simulink model "crossroad_cs_old"  (R2021a)
settings: Solver=ode5  StartTime=0.0  StopTime=50  FixedStep=1/1000  RelTol=1e-3
PreLoadFcn:
  | mbxruntime.callbacks.PreLoadFcn(bdroot);
PostLoadFcn:
  | mbxruntime.callbacks.PostLoadFcn(bdroot);
InitFcn:
  | mbxruntime.callbacks.InitFcn(bdroot);
StartFcn:
  | mbxruntime.callbacks.StartFcn(bdroot);
StopFcn:
  | mbxruntime.callbacks.StopFcn(bdroot);
model workspace: external: MAT-File .\crossroad_cs_hws.mat (data not in the file)
values from neighbouring files (symbols this model uses):
  c_factor = 43.75    [emplanner_init.m]
  cf = -175016    [emplanner_init.m]
  cr = -130634    [emplanner_init.m]
  KD_PID_distance = 0.0    (= 0)    [emplanner_init.m]
  KD_PID_speed = 0    [emplanner_init.m]
  KI_PID_distance = 0.0    (= 0)    [emplanner_init.m]
  KI_PID_speed = 0    [emplanner_init.m]
  KP_PID_distance = 0.5    [emplanner_init.m]
  KP_PID_speed = 1.8    [emplanner_init.m]
  la = 1.265    [emplanner_init.m]
  lb = 2.947-1.265    (= 1.682)    [emplanner_init.m]
  LQR_K1 = k(:,1)'    [emplanner_init.m]
  LQR_K2 = k(:,2)'    [emplanner_init.m]
  LQR_K3 = k(:,3)'    [emplanner_init.m]
  LQR_K4 = k(:,4)'    [emplanner_init.m]
  m = 2020    [emplanner_init.m]
  my_global_path_x = [0.4409 0.940746626271 1.44028225507 1.93950267328 2.43840536558 2.93698884522 3.43525224935 3.93319509352 4.43081712279 4.92811822143 5.42509835808 5.92175755256 ... (6001 elements, 6001x1)]    [my_global_path.mat]    (also in my_global_path_200.mat = [0.4409 0.940746626271 1.44028225507 1.93950267328 2.4384053)
  my_global_path_y = [58.2244 58.2243999975 58.2243999675 58.2243998683 58.224399668 58.2243993499 58.2243989099 58.2243983526 58.2243976886 58.2243969324 58.2243961011 58.2243952132 ... (6001 elements, 6001x1)]    [my_global_path.mat]    (also in my_global_path_200.mat = [58.2244 58.2243999975 58.2243999675 58.2243998683 58.224399)
  rack_displacement = [-39.14 , -37.2 , -35.29 , -33.43 , -31.6 , -29.81 , -28.06 , -26.34 , -24.66 ,      -23.01 , -21.38 , -19.79 , -18.23 , -16.69 , -15.18 , -13.7 , -12.23 , -10.8 , -9.38 , -7.98 ,     -6.61 , -5.25 , -3.91 , -2.59 , -1.29 , 0 , 1.27 , 2.54 , 3.78 , 5.02 , 6.24 , 7.46 , 8.66 ,      9.86 , 11.05 , 12.24 , 13.41 , 14.59 , 15.76 , 16.92 , 18.09 , 19.25 , 20.42 , 21.59 , 22.76 ,      23.93 , 25.11 , 26 ...(+26 chars)    [emplanner_init.m]
  right_wheel_ground = [-70 ,-67.2 , -64.4 , -61.6 , -58.8 , -56 , -53.2 , -50.4 , -47.6 , -44.8 , -42 ,      -39.2 , -36.4 , -33.6 , -30.8 , -28 , -25.2 , -22.4 , -19.6 , -16.8 , -14 , -11.2 , -8.4 , -5.6 ,      -2.8 , 0 , 2.8 , 5.6 , 8.4 , 11.2 , 14 , 16.8 , 19.6 , 22.4 , 25.2 , 28 , 30.8 , 33.6 , 36.4 ,      39.2 , 42 , 44.8 , 47.6 , 50.4 , 53.2 , 56 , 58.8 , 61.6 , 64.4 , 67.2 , 70 ]    [emplanner_init.m]
  vx_break_point = zeros(1,5000)    [emplanner_init.m]
undefined symbols (not defined in the file or in its folder): aubr, DiscIntNeverNeededParam, tablebr, vubr
libraries: PreScanSimulinkLibrary x11, Solver_SF x1
(part 2 of 8)

== system crossroad_cs_old/STATE_Box_4_bus ==
  STATE_Box_4_bus : Inport  Tag=inport/StatePort  OutDataTypeStr=Bus: PRESCAN_STATEACTUATORDATA  PortDimensions=1  SampleTime=50/1000  BusOutputAsStruct=on
  Actuator : S-Function  FunctionName=sfun_StateActuator  Parameters=UniqueID, TimeStep  SFunctionDeploymentMode=off  EnableBusSupport=off  mask(PreScan Sink Block: State){UniqueID=745, TimeStep=50/1000}
      mask prompts: UniqueID "Auto-Assigned: Unique ID"; TimeStep "Auto-Assigned: Upload Period [s]"
      mask help:
      | The Actor State contains a vector signal of size (9x1), containing the following signals:
      |
      | -  Position    	(x,y,z)             	[m]
      | -  Velocity    	(vx,vy,vz)         	[m/s]
      | -  Angles       	(Roll, Pitch, Yaw)	[rad]
      |
      | The Actor state is defined in the global axis system.
      | The state is superponed on the Initial position defined in the GUI.
      |
      | For more information, please click Help.
      mask Help: eval('openHelp(222)')
      mask Display: image(imread('State.png'))
  wires:
  STATE_Box_4_bus/1 -> Actuator/1

== system crossroad_cs_old/Synchronizer ==
  Bus Selector1 : BusSelector  OutputSignals=FederateStopped
  Stop Simulation : Stop
  sfun_Synchronizer : S-Function  FunctionName=sfun_Synchronizer  Parameters=SampleTime  SFunctionDeploymentMode=off  EnableBusSupport=off  mask(Legacy Function){SFunctionSpec=void prescan_synchronizer_outputFcn(void ** work1, PRESCAN_SYNCHRONIZEDATA y1[1]), SampleTime=TimeStep, ShowSpec=on}
      mask prompts: SampleTime "Sample time (-1 for inherited):"; ShowSpec "Display function specification"
      mask help:
      | This block allows you to call the legacy functions specified by the following Legacy Code Tool definition:
      | def.SFunctionName = 'sfun_Synchronizer';
      | def.OutputFcnSpec = 'void prescan_synchronizer_outputFcn(void ** work1, PRESCAN_SYNCHRONIZEDATA y1[1])';
      | def.StartFcnSpec = 'void prescan_synchronizer_startFcn(void ** work1)';
      | def.TerminateFcnSpec = 'void prescan_synchronizer_terminateFcn(void ** work1)';
      | def.HeaderFiles = {'prescan_synchronizer_data.h'};
      | def.HostLibFiles = {'sensorinterfaced.lib'};
      | def.IncPaths = {'src', 'C:\prescandev\vislibrary\vis\..\pimp\include\sensors\InterfaceRTW'};
      | def.SrcPaths = {'src'};
      | def.LibPaths = {'C:\\prescandev\\vislibrary_build\lib'};
      | def.SampleTime = 'parameterized';
      | def.Options.language = 'C';
      mask Help: <p>This block was generated automatically by the Legacy Code Tool. For detailed help on this tool, call<a href="matlab:legacy_code('help')"> legacy_code('help')</a>.</p>
      mask Callback ShowSpec:
      | if strcmp(get_param(gcbh, 'ShowSpec'), 'on')
      |   set_param(gcbh, 'MaskDisplay', sprintf('fprintf(''%s'');', get_param(gcbh, 'SFunctionSpec')));
      | else
      |   set_param(gcbh, 'MaskDisplay', sprintf('fprintf(''%s'');', get_param(gcbh, 'FunctionName')));
      | end
      mask Display: fprintf('void prescan_synchronizer_outputFcn(void ** work1, PRESCAN_SYNCHRONIZEDATA y1[1])');
  wires:
  Bus Selector1/1 -> Stop Simulation/1  "<FederateStopped>"
  sfun_Synchronizer/1 -> Bus Selector1/1

== system crossroad_cs_old/Audi_A8_Sedan_1/AIR_1_Demux ==
  AIR : Inport
  Activate_Switch : Subsystem
      mask Display: text(5,10,'')
  Bus Selector : BusSelector  OutputSignals=DATA.Range,DATA.Azimuth,DATA.Elevation,DATA.ID,DATA.Velocity,DATA.Heading
  Data Type Conversion : DataTypeConversion  OutDataTypeStr=double
  For Iterator : ForIterator  ResetStates=reset  IterationLimit=detectableObjects
  Selector : Selector  InputPortWidth=detectableObjects  IndexOptions=Index vector (port)  Indices=[1 3]  OutputSizes=1
  Signal2ArrayOfSignals1 : Subsystem  mask{VECTORLENGTH=detectableObjects}
      mask prompts: VECTORLENGTH "Length of vector"
  Signal2ArrayOfSignals2 : Subsystem  mask{VECTORLENGTH=detectableObjects}
      mask prompts: VECTORLENGTH "Length of vector"
  Signal2ArrayOfSignals3 : Subsystem  mask{VECTORLENGTH=detectableObjects}
      mask prompts: VECTORLENGTH "Length of vector"
  Signal2ArrayOfSignals4 : Subsystem  mask{VECTORLENGTH=detectableObjects}
      mask prompts: VECTORLENGTH "Length of vector"
  Signal2ArrayOfSignals5 : Subsystem  mask{VECTORLENGTH=detectableObjects}
      mask prompts: VECTORLENGTH "Length of vector"
  Signal2ArrayOfSignals6 : Subsystem  mask{VECTORLENGTH=detectableObjects}
      mask prompts: VECTORLENGTH "Length of vector"
  Range [m] : Outport
  Azimuth [deg] : Outport  Port=2
  Elevation [deg] : Outport  Port=3
  ID [-] : Outport  Port=4
  Velocity [m/s] : Outport  Port=5
  Heading [deg] : Outport  Port=6
  wires:
  Data Type Conversion/1 -> ID [-]/1
  Bus Selector/6 -> Signal2ArrayOfSignals6/2(Element)  "<Heading>"
  Signal2ArrayOfSignals6/1(ArrayofElements) -> Activate_Switch/2(Heading)
  Bus Selector/5 -> Signal2ArrayOfSignals5/2(Element)  "<Velocity>"
  Signal2ArrayOfSignals5/1(ArrayofElements) -> Velocity [m/s]/1
  Bus Selector/4 -> Signal2ArrayOfSignals4/2(Element)  "<ID>"
  Signal2ArrayOfSignals4/1(ArrayofElements) -> Data Type Conversion/1, Activate_Switch/1(BeamID)
  Bus Selector/3 -> Signal2ArrayOfSignals3/2(Element)  "<Elevation>"
  Signal2ArrayOfSignals3/1(ArrayofElements) -> Elevation [deg]/1
  Bus Selector/2 -> Signal2ArrayOfSignals1/2(Element)  "<Azimuth>"
  Signal2ArrayOfSignals1/1(ArrayofElements) -> Azimuth [deg]/1
  Signal2ArrayOfSignals2/1(ArrayofElements) -> Range [m]/1
  Bus Selector/1 -> Signal2ArrayOfSignals2/2(Element)  "<Range>"
  Selector/1 -> Bus Selector/1
  For Iterator/1 -> Signal2ArrayOfSignals6/1(LoopIndex), Signal2ArrayOfSignals5/1(LoopIndex), Signal2ArrayOfSignals4/1(LoopIndex), Signal2ArrayOfSignals3/1(LoopIndex), Signal2ArrayOfSignals1/1(LoopIndex), Signal2ArrayOfSignals2/1(LoopIndex), Selector/2
  AIR/1 -> Selector/1
  Activate_Switch/1(On/Off) -> Heading [deg]/1

== system crossroad_cs_old/Audi_A8_Sedan_1/Dynamics_UserSpecified ==
  note: For state mode 'Dynamic' positions
      | are not taken into account, as they
      | are computed by integrating velocity.
      | Click annotation for Help.
  steer_sw : Inport
  throttle : Inport  Port=2
  brake : Inport  Port=3
  CarSim S-Function2 : Solver_SF/CarSim S-Function  Priority=1  SIMFILE=D:\CARSIM2019.1\DynamicModel\simfile.sim
  CarSim2PreScanSTATE : Subsystem  Tag=CarSim2PreScanSTATE  mask(CarSim2PreScan:){z0=0}
      mask prompts: z0 "PreScan Actor initial COG z-position wrt GLOBAL axis system [m]"
      mask help: This block converts the outputs coming from the CarSim block into consistent PreScan signals.
  Constant : Constant  Value=ones(1,8)*1
  Ground : Ground
  Ground1 : Ground
  Mux : Mux  Inputs=[1 1 1 12 8]
  MuxState : Subsystem  Tag=mux/State  mask(Empty Dynamics State Block){positioningmode=on, TimeStep=1/1000}
      mask prompts: positioningmode "Positioning Mode"; TimeStep "Auto Assigned: Time Step [s]"
      mask help:
      | Build the state of an actor based on user input.
      | The user can either use positioning mode or dynamics mode.
      | - When using positioning mode the position and orientation of the actor are set directly based on the input. Expected input is relative to the initial position and orientation of the actor. It's also possible to specify the velocity of the actor, though this input isn't used, only passed on.
      | - When using dynamics mode the position input is ignored. Expected input is velocity and orientation. The velocity is relative the current orientation of the actor, while orientation is relative to its initial orientation. The position of the actor is calculated based on the velocity and orientation given.
      settings: DeleteFcn=PreScanBlockDeleteFcn;
  STATE_Audi_A8_Sedan_1 : Subsystem  Tag=mux/StatePort  Priority=0  LoadFcn=load PrescanStateActuatorData  mask(PreScan Sink Block: State){x0=3.6384, y0=57.8912, z0=0.55, Roll0=0, Pitch0=0, Yaw0=0, TimeStep=1/1000}
      mask prompts: x0 "Ini x-position VEHICLE wrt GLOBAL axis system [m]"; y0 "Ini y-position VEHICLE wrt GLOBAL axis system [m]"; z0 "Ini z-position VEHICLE wrt GLOBAL axis system [m]"; Roll0 "Ini roll-angle BODY wrt VEHICLE axis system [deg]"; Pitch0 "Ini pitch-angle BODY wrt VEHICLE axis system [deg]"; Yaw0 "Ini yaw-angle VEHICLE wrt GLOBAL axis system [deg]"; TimeStep "Auto-Assigned: Upload Period [s]"
      mask help:
      | The Actor State contains a vector signal of size (9x1), containing the following signals:
      |
      | -  Position                  (x,y,z)                                     [m]
      | -  Velocity                  (vx,vy,vz)                               [m/s]
      | -  Angles                    (Roll, Pitch, Yaw)                   [rad]
      |
      | The Actor state is defined in the global axis system.
      | The state is superponed on the Initial position defined in the GUI.
      |
      | For more information, please click Help.
      settings: DeleteFcn=PreScanBlockDeleteFcn;
      mask Help: eval('openHelp(222)')
      mask Display: image(imread('State.png'))
  Scope : Scope
  State : Outport
  vx : Outport  Port=2
  vy : Outport  Port=3
  ax : Outport  Port=4
  ay : Outport  Port=5
  wires:
  Ground/1 -> Mux/4
  brake/1 -> Mux/3
  steer_sw/1 -> Mux/1
  Constant/1 -> Mux/5
  throttle/1 -> Mux/2
  CarSim S-Function2/1 -> CarSim2PreScanSTATE/1(CarSim_In)
  CarSim2PreScanSTATE/7(R [rad]) -> MuxState/7(R [rad])
  CarSim2PreScanSTATE/9(Y [rad]) -> MuxState/9(Y [rad])
  CarSim2PreScanSTATE/11(ay[m/s^2]) -> ay/1
  CarSim2PreScanSTATE/2(y [m]) -> MuxState/2(y [m])
  CarSim2PreScanSTATE/6(dz [m/s]) -> MuxState/6(dz [m/s])
  CarSim2PreScanSTATE/10(ax[m/s^2]) -> ax/1
  CarSim2PreScanSTATE/1(x [m]) -> Scope/1, MuxState/1(x [m])
  CarSim2PreScanSTATE/4(dx [m/s]) -> vx/1, MuxState/4(dx [m/s])
  CarSim2PreScanSTATE/8(P [rad]) -> MuxState/8(P [rad])
  CarSim2PreScanSTATE/3(z [m]) -> MuxState/3(z [m])
  CarSim2PreScanSTATE/5(dy [m/s]) -> vy/1, MuxState/5(dy [m/s])
  MuxState/1(state) -> State/1, STATE_Audi_A8_Sedan_1/1(State)
  Mux/1 -> CarSim S-Function2/1
  Ground1/1 -> ?
  STATE_Audi_A8_Sedan_1/1(StateBus) -> ?

== system crossroad_cs_old/Audi_A8_Sedan_1/SELF_Demux ==
  SELF : Inport  OutDataTypeStr=Bus: PRESCAN_SELFSENSORDATA
  Bus Selector : BusSelector  OutputSignals=PositionX,PositionY,PositionZ,OrientationRoll,OrientationPitch,OrientationYaw,Velocity,Yaw_rate,Lat,Long,Alt
  Demux2 : Demux  Outputs=3
  Gain : Gain  Gain=180/pi
  Gain1 : Gain  Gain=180/pi
  Vector Concatenate1 : Concatenate  NumInputs=3
  compas converter : Subsystem
  x [m] : Outport
  y [m] : Outport  Port=2
  z [m] : Outport  Port=3
  rotx [deg] : Outport  Port=4
  roty [deg] : Outport  Port=5
  rotz [deg] : Outport  Port=6
  GPS lat [deg] : Outport  Port=7
  GPS long [deg] : Outport  Port=8
  GPS alt [m] : Outport  Port=9
  velocity [m/s] : Outport  Port=10
  heading [deg] : Outport  Port=11
  yaw rate [deg/s] : Outport  Port=12
  wires:
  Bus Selector/11 -> GPS alt [m]/1  "<Alt>"
  Bus Selector/10 -> GPS long [deg]/1  "<Long>"
  Bus Selector/9 -> GPS lat [deg]/1  "<Lat>"
  Bus Selector/8 -> Gain1/1  "<Yaw_rate>"
  Bus Selector/6 -> compas converter/1(rotz [rad]), Vector Concatenate1/3  "<OrientationYaw>"
  Bus Selector/5 -> Vector Concatenate1/2  "<OrientationPitch>"
  Bus Selector/4 -> Vector Concatenate1/1  "<OrientationRoll>"
  Vector Concatenate1/1 -> Gain/1
  Bus Selector/3 -> z [m]/1  "<PositionZ>"
  SELF/1 -> Bus Selector/1
  Gain/1 -> Demux2/1
  Demux2/1 -> rotx [deg]/1
  Demux2/2 -> roty [deg]/1
  Demux2/3 -> rotz [deg]/1
  compas converter/1(heading [deg]) -> heading [deg]/1
  Gain1/1 -> yaw rate [deg/s]/1
  Bus Selector/1 -> x [m]/1  "<PositionX>"
  Bus Selector/2 -> y [m]/1  "<PositionY>"
  Bus Selector/7 -> velocity [m/s]/1  "<Velocity>"

== system crossroad_cs_old/Audi_A8_Sedan_1/STATE_Audi_A8_Sedan_1 ==
  State : Inport  SampleTime=TimeStep
  Bus Creator : BusCreator  Inputs=15  OutDataTypeStr=Bus: PRESCAN_STATEACTUATORDATA  NonVirtualBus=on
  Constant : Constant  Value=0
  Demux : Demux  Outputs=15
  Mux : Mux  Inputs=3
  Mux1 : Mux  Inputs=3
  Mux2 : Mux  Inputs=3
  iniBODYAngles wrtVEH [rad] : Constant  Value=Roll0  SampleTime=TimeStep
  iniBODYAngles wrtVEH [rad]1 : Constant  Value=Pitch0  SampleTime=TimeStep
  iniVEHAngles wrtGLOB [rad] : Constant  Value=Yaw0  SampleTime=TimeStep
  iniVEHposition wrtGLOB [m] : Constant  Value=x0  SampleTime=TimeStep
  iniVEHposition wrtGLOB [m]1 : Constant  Value=y0  SampleTime=TimeStep
  iniVEHposition wrtGLOB [m]2 : Constant  Value=z0  SampleTime=TimeStep
  state2FullState : PreScanSimulinkLibrary/state2FullState  SystemSampleTime=-1  VariantActivationTime=update diagram  Latency=0  AutoFrameSizeCalculation=off
  StateBus : Outport  OutDataTypeStr=Bus: PRESCAN_STATEACTUATORDATA
  wires:
  Mux2/1 -> state2FullState/4
  iniVEHAngles wrtGLOB [rad]/1 -> Mux2/3
  Mux1/1 -> state2FullState/3
  Constant/1 -> Mux2/1, Mux2/2, Mux1/3
  iniBODYAngles wrtVEH [rad]1/1 -> Mux1/2
  iniBODYAngles wrtVEH [rad]/1 -> Mux1/1
  Mux/1 -> state2FullState/2
  iniVEHposition wrtGLOB [m]2/1 -> Mux/3
  iniVEHposition wrtGLOB [m]/1 -> Mux/1
  iniVEHposition wrtGLOB [m]1/1 -> Mux/2
  Demux/15 -> Bus Creator/15  "AngularVelocityYaw"
  Demux/14 -> Bus Creator/14  "AngularVelocityPitch"
  Demux/13 -> Bus Creator/13  "AngularVelocityRoll"
  Demux/12 -> Bus Creator/12  "OrientationYaw"
  Demux/11 -> Bus Creator/11  "OrientationPitch"
  Demux/10 -> Bus Creator/10  "OrientationRoll"
  Demux/9 -> Bus Creator/9  "AccelerationZ"
  Demux/8 -> Bus Creator/8  "AccelerationY"
  Demux/7 -> Bus Creator/7  "AccelerationX"
  Demux/6 -> Bus Creator/6  "VelocityZ"
  Demux/5 -> Bus Creator/5  "VelocityY"
  Demux/4 -> Bus Creator/4  "VelocityX"
  Demux/3 -> Bus Creator/3  "PositionZ"
  Demux/2 -> Bus Creator/2  "PositionY"
  Demux/1 -> Bus Creator/1  "PositionX"
  state2FullState/1 -> Demux/1
  State/1 -> state2FullState/1
  Bus Creator/1 -> StateBus/1

== system crossroad_cs_old/Audi_A8_Sedan_1/control module1 ==
  location_info : Inport
  planning_result : Inport  Port=2
  control_predict_time[s] : Inport  Port=3
  current_time : Inport  Port=4
  Trigger : TriggerPort  TriggerType=function-call  VariantControl=Variant  PortDimensions=1
  Bus Selector : BusSelector  OutputSignals=trajectory_x_gcs,trajectory_y_gcs,trajectory_heading_gcs,trajectory_kappa_gcs,trajectory_speed_gcs,trajectory_accel_gcs,trajectory_time_gcs
  Bus Selector1 : BusSelector  OutputSignals=host_x,host_y,host_heading_xy,host_vx,host_vy,host_yawrate,host_speed
  MATLAB Function : MATLAB Function  TreatAsAtomicUnit=on
  control main : Subsystem
  lateral_steer_sw : Outport
  throttle : Outport  Port=2
  brake : Outport  Port=3
  debug_control : Outport  Port=4
  wires:
  Bus Selector1/5 -> control main/5(host_vy[m/s])  "<host_vy>"
  Bus Selector1/4 -> control main/4(host_vx[m/s])  "<host_vx>"
  Bus Selector1/2 -> control main/2(host_y[m])  "<host_y>"
  Bus Selector1/7 -> control main/7(host_speed[m/s])  "<host_speed>"
  control main/2(throttle) -> throttle/1
  Bus Selector1/1 -> control main/1(host_x[m])  "<host_x>"
  Bus Selector1/6 -> control main/6(host_yawrate[rad/s])  "<host_yawrate>"
  Bus Selector1/3 -> control main/3(host_heading_xy[rad])  "<host_heading_xy>"
  location_info/1 -> Bus Selector1/1
  control_predict_time[s]/1 -> control main/14(control_predict_time[s])
  control main/4(debug_control) -> debug_control/1
  control main/1(lateral_steer_sw) -> lateral_steer_sw/1
  control main/3(brake) -> brake/1
  MATLAB Function/6(ar) -> control main/13(accelerate_desire[m/s^2])
  MATLAB Function/5(vr) -> control main/12(speed_desire[m/s])
  MATLAB Function/4(kappar) -> control main/11(kappar_desire[m^-1])
  MATLAB Function/3(thetar) -> control main/10(thetar_desire[rad])
  MATLAB Function/2(yr) -> control main/9(yr_desire[m])
  MATLAB Function/1(xr) -> control main/8(xr_desire[m])
  current_time/1 -> MATLAB Function/8(current_time)
  planning_result/1 -> Bus Selector/1
  Bus Selector/1 -> [trajecotory_x]  "<trajectory_x_gcs>"
  Bus Selector/2 -> [trajecotory_y]  "<trajectory_y_gcs>"
  Bus Selector/3 -> [trajecotory_heading]  "<trajectory_heading_gcs>"
  Bus Selector/4 -> [trajecotory_kappa]  "<trajectory_kappa_gcs>"
  Bus Selector/5 -> [trajecotory_speed]  "<trajectory_speed_gcs>"
  Bus Selector/6 -> [trajecotory_accel]  "<trajectory_accel_gcs>"
  Bus Selector/7 -> [trajecotory_time]  "<trajectory_time_gcs>"
  [trajecotory_time] -> MATLAB Function/7(trajectory_time)
  [trajecotory_accel] -> MATLAB Function/6(trajectory_accel)
  [trajecotory_speed] -> MATLAB Function/5(trajectory_speed)
  [trajecotory_kappa] -> MATLAB Function/4(trajectory_kappa)
  [trajecotory_heading] -> MATLAB Function/3(trajectory_heading)
  [trajecotory_y] -> MATLAB Function/2(trajectory_y)
  [trajecotory_x] -> MATLAB Function/1(trajectory_x)

== system crossroad_cs_old/Audi_A8_Sedan_1/decision&planning module ==
  location info : Inport
  routine info : Inport  Port=2
  perception info : Inport  Port=3
  pre planning info : Inport  Port=4
  current time : Inport  Port=5
  Trigger : TriggerPort  TriggerType=function-call  VariantControl=Variant  PortDimensions=1
  Bus Selector : BusSelector  OutputSignals=host_x,host_y,host_heading_xy,host_vx,host_vy,host_yawrate,host_speed
  Bus Selector1 : BusSelector  OutputSignals=referenceline_x,referenceline_y,referenceline_heading,referenceline_kappa
  EM Planner : Subsystem
  referenceline provider : Subsystem
  planning_result : Outport
  wires:
  [planning_result] -> planning_result/1
  routine info/1 -> referenceline provider/2(routine info)
  location info/1 -> EM Planner/2(location info), Bus Selector/1, referenceline provider/1(location info)
  Bus Selector/7 -> [host_speed]  "<host_speed>"
  Bus Selector/1 -> [host_x]  "<host_x>"
  Bus Selector/3 -> [host_heading_xy]  "<host_heading_xy>"
  Bus Selector/4 -> [host_vx]  "<host_vx>"
  Bus Selector/5 -> [host_vy]  "<host_vy>"
  Bus Selector/2 -> [host_y]  "<host_y>"
  Bus Selector/6 -> [host_yawrate]  "<host_yawrate>"
  referenceline provider/1(referenceline info) -> EM Planner/1(referenceline info), [referenceline_info]
  referenceline provider/2(debug referenceline) -> [debug_referenceline]
  [referenceline_info] -> Bus Selector1/1
  Bus Selector1/1 -> [referenceline_x]  "<referenceline_x>"
  Bus Selector1/2 -> [referenceline_y]  "<referenceline_y>"
  Bus Selector1/3 -> [referenceline_heading]  "<referenceline_heading>"
  Bus Selector1/4 -> [referenceline_kappa]  "<referenceline_kappa>"
  perception info/1 -> EM Planner/3(perception info)
  pre planning info/1 -> EM Planner/4(pre_planning info)
  current time/1 -> EM Planner/5(current time)
  EM Planner/1(EM Planner result) -> [planning_result]

== system crossroad_cs_old/Audi_A8_Sedan_1/location module ==
  host_x[m] : Inport
  host_y[m] : Inport  Port=2
  host_heading_xy[rad] : Inport  Port=3
  host_vx[m/s] : Inport  Port=4
  host_vy[m/s] : Inport  Port=5
  host_yawrate[rad/s] : Inport  Port=6
  host_speed[m/s] : Inport  Port=7
  host_ax[m/s2] : Inport  Port=8
  host_ay[m/s2] : Inport  Port=9
  Bus Creator : BusCreator  Inputs=9
  location info : Outport
  wires:
  host_yawrate[rad/s]/1 -> Bus Creator/6
  host_vy[m/s]/1 -> Bus Creator/5
  host_heading_xy[rad]/1 -> Bus Creator/3
  host_speed[m/s]/1 -> Bus Creator/7
  Bus Creator/1 -> location info/1
  host_y[m]/1 -> Bus Creator/2
  host_x[m]/1 -> Bus Creator/1
  host_vx[m/s]/1 -> Bus Creator/4
  host_ax[m/s2]/1 -> Bus Creator/8
  host_ay[m/s2]/1 -> Bus Creator/9

== system crossroad_cs_old/Audi_A8_Sedan_1/perception module ==
  location info : Inport
  obs range : Inport  Port=2
  obs theta : Inport  Port=3
  obs velocity : Inport  Port=4
  obs heading : Inport  Port=5
  Bus Creator : BusCreator  Inputs=4
  Bus Selector : BusSelector  OutputSignals=host_x,host_y,host_heading_xy
  MATLAB Function : MATLAB Function  TreatAsAtomicUnit=on
  perception info : Outport
  wires:
  location info/1 -> Bus Selector/1
  Bus Selector/1 -> [host_x]  "<host_x>"
  Bus Selector/2 -> [host_y]  "<host_y>"
  Bus Selector/3 -> [host_heading_xy]  "<host_heading_xy>"
  obs range/1 -> [obs_range]
  obs theta/1 -> [obs_theta]
  obs velocity/1 -> [obs_velocity]
  obs heading/1 -> [obs_heading]
  [host_x] -> MATLAB Function/1(host_x)
  [host_y] -> MATLAB Function/2(host_y)
  [host_heading_xy] -> MATLAB Function/3(host_heading_xy)
  [obs_range] -> MATLAB Function/4(obs_range)
  [obs_theta] -> MATLAB Function/5(obs_theta)
  [obs_velocity] -> MATLAB Function/6(obs_velocity)
  [obs_heading] -> MATLAB Function/7(obs_velocity_heading)
  MATLAB Function/1(obs_x_set_gcs) -> [obs_x_set_gcs]
  MATLAB Function/2(obs_y_set_gcs) -> [obs_y_set_gcs]
  MATLAB Function/3(obs_velocity_set_gcs) -> [obs_velocity_set_gcs]
  MATLAB Function/4(obs_heading_set_gcs) -> [obs_heading_set_gcs]
  Bus Creator/1 -> perception info/1
  [obs_x_set_gcs] -> Bus Creator/1  "obs_x_set_gcs"
  [obs_y_set_gcs] -> Bus Creator/2  "obs_y_set_gcs"
  [obs_velocity_set_gcs] -> Bus Creator/3  "obs_velocity_set_gcs"
  [obs_heading_set_gcs] -> Bus Creator/4  "obs_heading_set_gcs"

== system crossroad_cs_old/Audi_A8_Sedan_1/routine module ==
  Bus Creator : BusCreator  Inputs=2
  Constant : Constant  Value=my_global_path_x
  Constant1 : Constant  Value=my_global_path_y
  global_path_info : Outport
  wires:
  Constant1/1 -> [global_path_y]
  Constant/1 -> [global_path_x]
  [global_path_x] -> Bus Creator/1  "global_path_x"
  [global_path_y] -> Bus Creator/2  "global_path_y"
  Bus Creator/1 -> global_path_info/1

== system crossroad_cs_old/Box_1/Dynamics_Empty ==
  note: For state mode 'Dynamic' positions
      | are not taken into account, as they
      | are computed by integrating velocity.
      | Click annotation for Help.
  Ground_{1..9} (9 alike) : Ground
  MuxState : Subsystem  Tag=mux/State  mask(Empty Dynamics State Block){positioningmode=on, TimeStep=1/1000}
      mask prompts: positioningmode "Positioning Mode"; TimeStep "Auto Assigned: Time Step [s]"
      mask help:
      | Build the state of an actor based on user input.
      | The user can either use positioning mode or dynamics mode.
      | - When using positioning mode the position and orientation of the actor are set directly based on the input. Expected input is relative to the initial position and orientation of the actor. It's also possible to specify the velocity of the actor, though this input isn't used, only passed on.
      | - When using dynamics mode the position input is ignored. Expected input is velocity and orientation. The velocity is relative the current orientation of the actor, while orientation is relative to its initial orientation. The position of the actor is calculated based on the velocity and orientation given.
      settings: DeleteFcn=PreScanBlockDeleteFcn;
  STATE_Box_1 : Subsystem  Tag=mux/StatePort  Priority=0  LoadFcn=load PrescanStateActuatorData  mask(PreScan Sink Block: State){x0=97.4125, y0=55.7557, z0=0.5, Roll0=0, Pitch0=0, Yaw0=0, TimeStep=1/1000}
      mask prompts: x0 "Ini x-position VEHICLE wrt GLOBAL axis system [m]"; y0 "Ini y-position VEHICLE wrt GLOBAL axis system [m]"; z0 "Ini z-position VEHICLE wrt GLOBAL axis system [m]"; Roll0 "Ini roll-angle BODY wrt VEHICLE axis system [deg]"; Pitch0 "Ini pitch-angle BODY wrt VEHICLE axis system [deg]"; Yaw0 "Ini yaw-angle VEHICLE wrt GLOBAL axis system [deg]"; TimeStep "Auto-Assigned: Upload Period [s]"
      mask help:
      | The Actor State contains a vector signal of size (9x1), containing the following signals:
      |
      | -  Position                  (x,y,z)                                     [m]
      | -  Velocity                  (vx,vy,vz)                               [m/s]
      | -  Angles                    (Roll, Pitch, Yaw)                   [rad]
      |
      | The Actor state is defined in the global axis system.
      | The state is superponed on the Initial position defined in the GUI.
      |
      | For more information, please click Help.
      settings: DeleteFcn=PreScanBlockDeleteFcn;
      mask Help: eval('openHelp(222)')
      mask Display: image(imread('State.png'))
  State : Outport  Tag=outport/StateOutport  SampleTime=1/1000
  wires:
  MuxState/1(state) -> STATE_Box_1/1(State)
  STATE_Box_1/1(StateBus) -> State/1
  Ground_1/1 -> MuxState/1(x [m])
  Ground_2/1 -> MuxState/2(y [m])
  Ground_3/1 -> MuxState/3(z [m])
  Ground_4/1 -> MuxState/4(dx [m/s])
  Ground_5/1 -> MuxState/5(dy [m/s])
  Ground_6/1 -> MuxState/6(dz [m/s])
  Ground_7/1 -> MuxState/7(R [rad])
  Ground_8/1 -> MuxState/8(P [rad])
  Ground_9/1 -> MuxState/9(Y [rad])

== system crossroad_cs_old/Box_1/SELF_Demux ==
  SELF : Inport  OutDataTypeStr=Bus: PRESCAN_SELFSENSORDATA
  Bus Selector : BusSelector  OutputSignals=PositionX,PositionY,PositionZ,OrientationRoll,OrientationPitch,OrientationYaw,Velocity,Yaw_rate,Lat,Long,Alt
  Demux2 : Demux  Outputs=3
  Gain : Gain  Gain=180/pi
  Gain1 : Gain  Gain=180/pi
  Vector Concatenate1 : Concatenate  NumInputs=3
  compas converter : Subsystem
  x [m] : Outport
  y [m] : Outport  Port=2
  z [m] : Outport  Port=3
  rotx [deg] : Outport  Port=4
  roty [deg] : Outport  Port=5
  rotz [deg] : Outport  Port=6
  GPS lat [deg] : Outport  Port=7
  GPS long [deg] : Outport  Port=8
  GPS alt [m] : Outport  Port=9
  velocity [m/s] : Outport  Port=10
  heading [deg] : Outport  Port=11
  yaw rate [deg/s] : Outport  Port=12
  wires:
  Bus Selector/11 -> GPS alt [m]/1  "<Alt>"
  Bus Selector/10 -> GPS long [deg]/1  "<Long>"
  Bus Selector/9 -> GPS lat [deg]/1  "<Lat>"
  Bus Selector/8 -> Gain1/1  "<Yaw_rate>"
  Bus Selector/7 -> velocity [m/s]/1  "<Velocity>"
  Bus Selector/6 -> compas converter/1(rotz [rad]), Vector Concatenate1/3  "<OrientationYaw>"
  Bus Selector/5 -> Vector Concatenate1/2  "<OrientationPitch>"
  Bus Selector/4 -> Vector Concatenate1/1  "<OrientationRoll>"
  Vector Concatenate1/1 -> Gain/1
  Bus Selector/3 -> z [m]/1  "<PositionZ>"
  Bus Selector/2 -> y [m]/1  "<PositionY>"
  Bus Selector/1 -> x [m]/1  "<PositionX>"
  SELF/1 -> Bus Selector/1
  Gain/1 -> Demux2/1
  Demux2/1 -> rotx [deg]/1
  Demux2/2 -> roty [deg]/1
  Demux2/3 -> rotz [deg]/1
  compas converter/1(heading [deg]) -> heading [deg]/1
  Gain1/1 -> yaw rate [deg/s]/1

== system crossroad_cs_old/Box_2/Dynamics_Empty ==
  note: For state mode 'Dynamic' positions
      | are not taken into account, as they
      | are computed by integrating velocity.
      | Click annotation for Help.
  Ground_{1..9} (9 alike) : Ground
  MuxState : Subsystem  Tag=mux/State  mask(Empty Dynamics State Block){positioningmode=on, TimeStep=1/1000}
      mask prompts: positioningmode "Positioning Mode"; TimeStep "Auto Assigned: Time Step [s]"
      mask help:
      | Build the state of an actor based on user input.
      | The user can either use positioning mode or dynamics mode.
      | - When using positioning mode the position and orientation of the actor are set directly based on the input. Expected input is relative to the initial position and orientation of the actor. It's also possible to specify the velocity of the actor, though this input isn't used, only passed on.
      | - When using dynamics mode the position input is ignored. Expected input is velocity and orientation. The velocity is relative the current orientation of the actor, while orientation is relative to its initial orientation. The position of the actor is calculated based on the velocity and orientation given.
      settings: DeleteFcn=PreScanBlockDeleteFcn;
  STATE_Box_2 : Subsystem  Tag=mux/StatePort  Priority=0  LoadFcn=load PrescanStateActuatorData  mask(PreScan Sink Block: State){x0=131.1114, y0=61.7864, z0=0.5, Roll0=0, Pitch0=0, Yaw0=0, TimeStep=1/1000}
      mask prompts: x0 "Ini x-position VEHICLE wrt GLOBAL axis system [m]"; y0 "Ini y-position VEHICLE wrt GLOBAL axis system [m]"; z0 "Ini z-position VEHICLE wrt GLOBAL axis system [m]"; Roll0 "Ini roll-angle BODY wrt VEHICLE axis system [deg]"; Pitch0 "Ini pitch-angle BODY wrt VEHICLE axis system [deg]"; Yaw0 "Ini yaw-angle VEHICLE wrt GLOBAL axis system [deg]"; TimeStep "Auto-Assigned: Upload Period [s]"
      mask help:
      | The Actor State contains a vector signal of size (9x1), containing the following signals:
      |
      | -  Position                  (x,y,z)                                     [m]
      | -  Velocity                  (vx,vy,vz)                               [m/s]
      | -  Angles                    (Roll, Pitch, Yaw)                   [rad]
      |
      | The Actor state is defined in the global axis system.
      | The state is superponed on the Initial position defined in the GUI.
      |
      | For more information, please click Help.
      settings: DeleteFcn=PreScanBlockDeleteFcn;
      mask Help: eval('openHelp(222)')
      mask Display: image(imread('State.png'))
  State : Outport  Tag=outport/StateOutport  SampleTime=1/1000
  wires:
  MuxState/1(state) -> STATE_Box_2/1(State)
  STATE_Box_2/1(StateBus) -> State/1
  Ground_1/1 -> MuxState/1(x [m])
  Ground_2/1 -> MuxState/2(y [m])
  Ground_3/1 -> MuxState/3(z [m])
  Ground_4/1 -> MuxState/4(dx [m/s])
  Ground_5/1 -> MuxState/5(dy [m/s])
  Ground_6/1 -> MuxState/6(dz [m/s])
  Ground_7/1 -> MuxState/7(R [rad])
  Ground_8/1 -> MuxState/8(P [rad])
  Ground_9/1 -> MuxState/9(Y [rad])

== system crossroad_cs_old/Box_2/SELF_Demux ==
  SELF : Inport  OutDataTypeStr=Bus: PRESCAN_SELFSENSORDATA
  Bus Selector : BusSelector  OutputSignals=PositionX,PositionY,PositionZ,OrientationRoll,OrientationPitch,OrientationYaw,Velocity,Yaw_rate,Lat,Long,Alt
  Demux2 : Demux  Outputs=3
  Gain : Gain  Gain=180/pi
  Gain1 : Gain  Gain=180/pi
  Vector Concatenate1 : Concatenate  NumInputs=3
  compas converter : Subsystem
  x [m] : Outport
  y [m] : Outport  Port=2
  z [m] : Outport  Port=3
  rotx [deg] : Outport  Port=4
  roty [deg] : Outport  Port=5
  rotz [deg] : Outport  Port=6
  GPS lat [deg] : Outport  Port=7
  GPS long [deg] : Outport  Port=8
  GPS alt [m] : Outport  Port=9
  velocity [m/s] : Outport  Port=10
  heading [deg] : Outport  Port=11
  yaw rate [deg/s] : Outport  Port=12
  wires:
  Bus Selector/11 -> GPS alt [m]/1  "<Alt>"
  Bus Selector/10 -> GPS long [deg]/1  "<Long>"
  Bus Selector/9 -> GPS lat [deg]/1  "<Lat>"
  Bus Selector/8 -> Gain1/1  "<Yaw_rate>"
  Bus Selector/7 -> velocity [m/s]/1  "<Velocity>"
  Bus Selector/6 -> compas converter/1(rotz [rad]), Vector Concatenate1/3  "<OrientationYaw>"
  Bus Selector/5 -> Vector Concatenate1/2  "<OrientationPitch>"
  Bus Selector/4 -> Vector Concatenate1/1  "<OrientationRoll>"
  Vector Concatenate1/1 -> Gain/1
  Bus Selector/3 -> z [m]/1  "<PositionZ>"
  Bus Selector/2 -> y [m]/1  "<PositionY>"
  Bus Selector/1 -> x [m]/1  "<PositionX>"
  SELF/1 -> Bus Selector/1
  Gain/1 -> Demux2/1
  Demux2/1 -> rotx [deg]/1
  Demux2/2 -> roty [deg]/1
  Demux2/3 -> rotz [deg]/1
  compas converter/1(heading [deg]) -> heading [deg]/1
  Gain1/1 -> yaw rate [deg/s]/1

== system crossroad_cs_old/Box_3/Dynamics_Empty ==
  note: For state mode 'Dynamic' positions
      | are not taken into account, as they
      | are computed by integrating velocity.
      | Click annotation for Help.
  Ground_{1..9} (9 alike) : Ground
  MuxState : Subsystem  Tag=mux/State  mask(Empty Dynamics State Block){positioningmode=on, TimeStep=1/1000}
      mask prompts: positioningmode "Positioning Mode"; TimeStep "Auto Assigned: Time Step [s]"
      mask help:
      | Build the state of an actor based on user input.
      | The user can either use positioning mode or dynamics mode.
      | - When using positioning mode the position and orientation of the actor are set directly based on the input. Expected input is relative to the initial position and orientation of the actor. It's also possible to specify the velocity of the actor, though this input isn't used, only passed on.
      | - When using dynamics mode the position input is ignored. Expected input is velocity and orientation. The velocity is relative the current orientation of the actor, while orientation is relative to its initial orientation. The position of the actor is calculated based on the velocity and orientation given.
      settings: DeleteFcn=PreScanBlockDeleteFcn;
  STATE_Box_3 : Subsystem  Tag=mux/StatePort  Priority=0  LoadFcn=load PrescanStateActuatorData  mask(PreScan Sink Block: State){x0=167.6101, y0=55.6248, z0=0.5, Roll0=0, Pitch0=0, Yaw0=0, TimeStep=1/1000}
      mask prompts: x0 "Ini x-position VEHICLE wrt GLOBAL axis system [m]"; y0 "Ini y-position VEHICLE wrt GLOBAL axis system [m]"; z0 "Ini z-position VEHICLE wrt GLOBAL axis system [m]"; Roll0 "Ini roll-angle BODY wrt VEHICLE axis system [deg]"; Pitch0 "Ini pitch-angle BODY wrt VEHICLE axis system [deg]"; Yaw0 "Ini yaw-angle VEHICLE wrt GLOBAL axis system [deg]"; TimeStep "Auto-Assigned: Upload Period [s]"
      mask help:
      | The Actor State contains a vector signal of size (9x1), containing the following signals:
      |
      | -  Position                  (x,y,z)                                     [m]
      | -  Velocity                  (vx,vy,vz)                               [m/s]
      | -  Angles                    (Roll, Pitch, Yaw)                   [rad]
      |
      | The Actor state is defined in the global axis system.
      | The state is superponed on the Initial position defined in the GUI.
      |
      | For more information, please click Help.
      settings: DeleteFcn=PreScanBlockDeleteFcn;
      mask Help: eval('openHelp(222)')
      mask Display: image(imread('State.png'))
  State : Outport  Tag=outport/StateOutport  SampleTime=1/1000
  wires:
  MuxState/1(state) -> STATE_Box_3/1(State)
  STATE_Box_3/1(StateBus) -> State/1
  Ground_1/1 -> MuxState/1(x [m])
  Ground_2/1 -> MuxState/2(y [m])
  Ground_3/1 -> MuxState/3(z [m])
  Ground_4/1 -> MuxState/4(dx [m/s])
  Ground_5/1 -> MuxState/5(dy [m/s])
  Ground_6/1 -> MuxState/6(dz [m/s])
  Ground_7/1 -> MuxState/7(R [rad])
  Ground_8/1 -> MuxState/8(P [rad])
  Ground_9/1 -> MuxState/9(Y [rad])

== system crossroad_cs_old/Box_3/SELF_Demux ==
  SELF : Inport  OutDataTypeStr=Bus: PRESCAN_SELFSENSORDATA
  Bus Selector : BusSelector  OutputSignals=PositionX,PositionY,PositionZ,OrientationRoll,OrientationPitch,OrientationYaw,Velocity,Yaw_rate,Lat,Long,Alt
  Demux2 : Demux  Outputs=3
  Gain : Gain  Gain=180/pi
  Gain1 : Gain  Gain=180/pi
  Vector Concatenate1 : Concatenate  NumInputs=3
  compas converter : Subsystem
  x [m] : Outport
  y [m] : Outport  Port=2
  z [m] : Outport  Port=3
  rotx [deg] : Outport  Port=4
  roty [deg] : Outport  Port=5
  rotz [deg] : Outport  Port=6
  GPS lat [deg] : Outport  Port=7
  GPS long [deg] : Outport  Port=8
  GPS alt [m] : Outport  Port=9
  velocity [m/s] : Outport  Port=10
  heading [deg] : Outport  Port=11
  yaw rate [deg/s] : Outport  Port=12
  wires:
  Bus Selector/11 -> GPS alt [m]/1  "<Alt>"
  Bus Selector/10 -> GPS long [deg]/1  "<Long>"
  Bus Selector/9 -> GPS lat [deg]/1  "<Lat>"
  Bus Selector/8 -> Gain1/1  "<Yaw_rate>"
  Bus Selector/7 -> velocity [m/s]/1  "<Velocity>"
  Bus Selector/6 -> compas converter/1(rotz [rad]), Vector Concatenate1/3  "<OrientationYaw>"
  Bus Selector/5 -> Vector Concatenate1/2  "<OrientationPitch>"
  Bus Selector/4 -> Vector Concatenate1/1  "<OrientationRoll>"
  Vector Concatenate1/1 -> Gain/1
  Bus Selector/3 -> z [m]/1  "<PositionZ>"
  Bus Selector/2 -> y [m]/1  "<PositionY>"
  Bus Selector/1 -> x [m]/1  "<PositionX>"
  SELF/1 -> Bus Selector/1
  Gain/1 -> Demux2/1
  Demux2/1 -> rotx [deg]/1
  Demux2/2 -> roty [deg]/1
  Demux2/3 -> rotz [deg]/1
  compas converter/1(heading [deg]) -> heading [deg]/1
  Gain1/1 -> yaw rate [deg/s]/1

== system crossroad_cs_old/Box_4/Dynamics_Empty ==
  note: For state mode 'Dynamic' positions
      | are not taken into account, as they
      | are computed by integrating velocity.
      | Click annotation for Help.
  Ground_{1..9} (9 alike) : Ground
  MuxState : Subsystem  Tag=mux/State  mask(Empty Dynamics State Block){positioningmode=on, TimeStep=1/1000}
      mask prompts: positioningmode "Positioning Mode"; TimeStep "Auto Assigned: Time Step [s]"
      mask help:
      | Build the state of an actor based on user input.
      | The user can either use positioning mode or dynamics mode.
      | - When using positioning mode the position and orientation of the actor are set directly based on the input. Expected input is relative to the initial position and orientation of the actor. It's also possible to specify the velocity of the actor, though this input isn't used, only passed on.
      | - When using dynamics mode the position input is ignored. Expected input is velocity and orientation. The velocity is relative the current orientation of the actor, while orientation is relative to its initial orientation. The position of the actor is calculated based on the velocity and orientation given.
      settings: DeleteFcn=PreScanBlockDeleteFcn;
  STATE_Box_4 : Subsystem  Tag=mux/StatePort  Priority=0  LoadFcn=load PrescanStateActuatorData  mask(PreScan Sink Block: State){x0=203.6167, y0=62.1811, z0=0.5, Roll0=0, Pitch0=0, Yaw0=0, TimeStep=1/1000}
      mask prompts: x0 "Ini x-position VEHICLE wrt GLOBAL axis system [m]"; y0 "Ini y-position VEHICLE wrt GLOBAL axis system [m]"; z0 "Ini z-position VEHICLE wrt GLOBAL axis system [m]"; Roll0 "Ini roll-angle BODY wrt VEHICLE axis system [deg]"; Pitch0 "Ini pitch-angle BODY wrt VEHICLE axis system [deg]"; Yaw0 "Ini yaw-angle VEHICLE wrt GLOBAL axis system [deg]"; TimeStep "Auto-Assigned: Upload Period [s]"
      mask help:
      | The Actor State contains a vector signal of size (9x1), containing the following signals:
      |
      | -  Position                  (x,y,z)                                     [m]
      | -  Velocity                  (vx,vy,vz)                               [m/s]
      | -  Angles                    (Roll, Pitch, Yaw)                   [rad]
      |
      | The Actor state is defined in the global axis system.
      | The state is superponed on the Initial position defined in the GUI.
      |
      | For more information, please click Help.
      settings: DeleteFcn=PreScanBlockDeleteFcn;
      mask Help: eval('openHelp(222)')
      mask Display: image(imread('State.png'))
  State : Outport  Tag=outport/StateOutport  SampleTime=1/1000
  wires:
  MuxState/1(state) -> STATE_Box_4/1(State)
  STATE_Box_4/1(StateBus) -> State/1
  Ground_1/1 -> MuxState/1(x [m])
  Ground_2/1 -> MuxState/2(y [m])
  Ground_3/1 -> MuxState/3(z [m])
  Ground_4/1 -> MuxState/4(dx [m/s])
  Ground_5/1 -> MuxState/5(dy [m/s])
  Ground_6/1 -> MuxState/6(dz [m/s])
  Ground_7/1 -> MuxState/7(R [rad])
  Ground_8/1 -> MuxState/8(P [rad])
  Ground_9/1 -> MuxState/9(Y [rad])

== system crossroad_cs_old/Box_4/SELF_Demux ==
  SELF : Inport  OutDataTypeStr=Bus: PRESCAN_SELFSENSORDATA
  Bus Selector : BusSelector  OutputSignals=PositionX,PositionY,PositionZ,OrientationRoll,OrientationPitch,OrientationYaw,Velocity,Yaw_rate,Lat,Long,Alt
  Demux2 : Demux  Outputs=3
  Gain : Gain  Gain=180/pi
  Gain1 : Gain  Gain=180/pi
  Vector Concatenate1 : Concatenate  NumInputs=3
  compas converter : Subsystem
  x [m] : Outport
  y [m] : Outport  Port=2
  z [m] : Outport  Port=3
  rotx [deg] : Outport  Port=4
  roty [deg] : Outport  Port=5
  rotz [deg] : Outport  Port=6
  GPS lat [deg] : Outport  Port=7
  GPS long [deg] : Outport  Port=8
  GPS alt [m] : Outport  Port=9
  velocity [m/s] : Outport  Port=10
  heading [deg] : Outport  Port=11
  yaw rate [deg/s] : Outport  Port=12
  wires:
  Bus Selector/11 -> GPS alt [m]/1  "<Alt>"
  Bus Selector/10 -> GPS long [deg]/1  "<Long>"
  Bus Selector/9 -> GPS lat [deg]/1  "<Lat>"
  Bus Selector/8 -> Gain1/1  "<Yaw_rate>"
  Bus Selector/7 -> velocity [m/s]/1  "<Velocity>"
  Bus Selector/6 -> compas converter/1(rotz [rad]), Vector Concatenate1/3  "<OrientationYaw>"
  Bus Selector/5 -> Vector Concatenate1/2  "<OrientationPitch>"
  Bus Selector/4 -> Vector Concatenate1/1  "<OrientationRoll>"
  Vector Concatenate1/1 -> Gain/1
  Bus Selector/3 -> z [m]/1  "<PositionZ>"
  Bus Selector/2 -> y [m]/1  "<PositionY>"
  Bus Selector/1 -> x [m]/1  "<PositionX>"
  SELF/1 -> Bus Selector/1
  Gain/1 -> Demux2/1
  Demux2/1 -> rotx [deg]/1
  Demux2/2 -> roty [deg]/1
  Demux2/3 -> rotz [deg]/1
  compas converter/1(heading [deg]) -> heading [deg]/1
  Gain1/1 -> yaw rate [deg/s]/1

== system crossroad_cs_old/Audi_A8_Sedan_1/AIR_1_Demux/Activate_Switch ==
  BeamID : Inport
  Heading : Inport  Port=2
  Constant : Constant  Value=0
  Product1 : Product  RndMeth=Zero
  Relational Operator : RelationalOperator  Operator=~=  OutDataTypeStr=boolean  RndMeth=Nearest
  On/Off : Outport
  wires:
  Constant/1 -> Relational Operator/1
  Relational Operator/1 -> Product1/1
  BeamID/1 -> Relational Operator/2
  Product1/1 -> On/Off/1
  Heading/1 -> Product1/2

== system crossroad_cs_old/Audi_A8_Sedan_1/AIR_1_Demux/Signal2ArrayOfSignals1 ==
  note: Set mask parameter VECTORLENGTH
      |  to MAXMESSAGES
  note: Initial state of Previous vector block
      | set to zeros(VECTORLENGTH,1)
  LoopIndex : Inport
  Element : Inport  Port=2
  Assignment : Assignment  IndexOptions=Index vector (port)  Indices=1  OutputSizes=1
  Previous vector : Memory  InitialCondition=zeros(VECTORLENGTH,1)  InheritSampleTime=on
  ArrayofElements : Outport
  wires:
  Element/1 -> Assignment/2
  LoopIndex/1 -> Assignment/3
  Previous vector/1 -> Assignment/1
  Assignment/1 -> ArrayofElements/1, Previous vector/1

== system crossroad_cs_old/Audi_A8_Sedan_1/AIR_1_Demux/Signal2ArrayOfSignals2 ==
  note: Set mask parameter VECTORLENGTH
      |  to MAXMESSAGES
  note: Initial state of Previous vector block
      | set to zeros(VECTORLENGTH,1)
  LoopIndex : Inport
  Element : Inport  Port=2
  Assignment : Assignment  IndexOptions=Index vector (port)  Indices=1  OutputSizes=1
  Previous vector : Memory  InitialCondition=zeros(VECTORLENGTH,1)  InheritSampleTime=on
  ArrayofElements : Outport
  wires:
  Element/1 -> Assignment/2
  LoopIndex/1 -> Assignment/3
  Previous vector/1 -> Assignment/1
  Assignment/1 -> ArrayofElements/1, Previous vector/1

== system crossroad_cs_old/Audi_A8_Sedan_1/AIR_1_Demux/Signal2ArrayOfSignals3 ==
  note: Set mask parameter VECTORLENGTH
      |  to MAXMESSAGES
  note: Initial state of Previous vector block
      | set to zeros(VECTORLENGTH,1)
  LoopIndex : Inport
  Element : Inport  Port=2
  Assignment : Assignment  IndexOptions=Index vector (port)  Indices=1  OutputSizes=1
  Previous vector : Memory  InitialCondition=zeros(VECTORLENGTH,1)  InheritSampleTime=on
  ArrayofElements : Outport
  wires:
  Element/1 -> Assignment/2
  LoopIndex/1 -> Assignment/3
  Previous vector/1 -> Assignment/1
  Assignment/1 -> ArrayofElements/1, Previous vector/1

== system crossroad_cs_old/Audi_A8_Sedan_1/AIR_1_Demux/Signal2ArrayOfSignals4 ==
  note: Set mask parameter VECTORLENGTH
      |  to MAXMESSAGES
  note: Initial state of Previous vector block
      | set to zeros(VECTORLENGTH,1)
  LoopIndex : Inport
  Element : Inport  Port=2
  Assignment : Assignment  IndexOptions=Index vector (port)  Indices=1  OutputSizes=1
  Previous vector : Memory  InitialCondition=zeros(VECTORLENGTH,1)  InheritSampleTime=on
  ArrayofElements : Outport
  wires:
  Element/1 -> Assignment/2
  LoopIndex/1 -> Assignment/3
  Previous vector/1 -> Assignment/1
  Assignment/1 -> ArrayofElements/1, Previous vector/1

== system crossroad_cs_old/Audi_A8_Sedan_1/AIR_1_Demux/Signal2ArrayOfSignals5 ==
  note: Set mask parameter VECTORLENGTH
      |  to MAXMESSAGES
  note: Initial state of Previous vector block
      | set to zeros(VECTORLENGTH,1)
  LoopIndex : Inport
  Element : Inport  Port=2
  Assignment : Assignment  IndexOptions=Index vector (port)  Indices=1  OutputSizes=1
  Previous vector : Memory  InitialCondition=zeros(VECTORLENGTH,1)  InheritSampleTime=on
  ArrayofElements : Outport
  wires:
  Element/1 -> Assignment/2
  LoopIndex/1 -> Assignment/3
  Previous vector/1 -> Assignment/1
  Assignment/1 -> ArrayofElements/1, Previous vector/1

== system crossroad_cs_old/Audi_A8_Sedan_1/AIR_1_Demux/Signal2ArrayOfSignals6 ==
  note: Set mask parameter VECTORLENGTH
      |  to MAXMESSAGES
  note: Initial state of Previous vector block
      | set to zeros(VECTORLENGTH,1)
  LoopIndex : Inport
  Element : Inport  Port=2
  Assignment : Assignment  IndexOptions=Index vector (port)  Indices=1  OutputSizes=1
  Previous vector : Memory  InitialCondition=zeros(VECTORLENGTH,1)  InheritSampleTime=on
  ArrayofElements : Outport
  wires:
  Element/1 -> Assignment/2
  LoopIndex/1 -> Assignment/3
  Previous vector/1 -> Assignment/1
  Assignment/1 -> ArrayofElements/1, Previous vector/1

== system crossroad_cs_old/Audi_A8_Sedan_1/Dynamics_UserSpecified/CarSim2PreScanSTATE ==
  CarSim_In : Inport
  D2R : Gain  Gain=pi/180
  Demux : Demux  Outputs=[3 3 3 -1]
  Demux1 : Demux  Outputs=3
  Demux2 : Demux  Outputs=3
  Demux3 : Demux  Outputs=3
  Demux4 : Demux  Outputs=28
  Gain : Gain  Gain=9.8
  Gain1 : Gain  Gain=9.8
  Terminator_{1..26} (26 alike) : Terminator
  Transformation_SprungMassCarSim2PreScan : Subsystem
  km|h_to_m|s : Gain  Gain=1/3.6
  x [m] : Outport
  y [m] : Outport  Port=2
  z [m] : Outport  Port=3
  dx [m/s] : Outport  Port=4
  dy [m/s] : Outport  Port=5
  dz [m/s] : Outport  Port=6
  R [rad] : Outport  Port=7
  P [rad] : Outport  Port=8
  Y [rad] : Outport  Port=9
  ax[m/s^2] : Outport  Port=10
  ay[m/s^2] : Outport  Port=11
  wires:
  Demux/4 -> Demux4/1
  Demux3/3 -> Y [rad]/1
  Demux3/2 -> P [rad]/1
  Demux3/1 -> R [rad]/1
  Demux2/3 -> dz [m/s]/1
  Demux2/2 -> dy [m/s]/1
  Demux2/1 -> dx [m/s]/1
  Demux1/3 -> z [m]/1
  Demux1/2 -> y [m]/1
  Demux1/1 -> x [m]/1
  Transformation_SprungMassCarSim2PreScan/1(Out1) -> Demux1/1
  Demux/1 -> Transformation_SprungMassCarSim2PreScan/1(In1)
  CarSim_In/1 -> Demux/1
  km|h_to_m|s/1 -> Demux2/1
  Demux/2 -> km|h_to_m|s/1
  Demux/3 -> D2R/1
  D2R/1 -> Demux3/1
  Demux4/28 -> Gain1/1
  Demux4/27 -> Gain/1
  Gain/1 -> ax[m/s^2]/1
  Gain1/1 -> ay[m/s^2]/1
  Demux4/1 -> Terminator_1/1
  Demux4/2 -> Terminator_2/1
  Demux4/3 -> Terminator_3/1
  Demux4/4 -> Terminator_4/1
  Demux4/5 -> Terminator_5/1
  Demux4/6 -> Terminator_6/1
  Demux4/7 -> Terminator_7/1
  Demux4/8 -> Terminator_8/1
  Demux4/9 -> Terminator_9/1
  Demux4/10 -> Terminator_10/1
  Demux4/11 -> Terminator_11/1
  Demux4/12 -> Terminator_12/1
  Demux4/13 -> Terminator_13/1
  Demux4/14 -> Terminator_14/1
  Demux4/15 -> Terminator_15/1
  Demux4/16 -> Terminator_16/1
  Demux4/17 -> Terminator_17/1
  Demux4/18 -> Terminator_18/1
  Demux4/19 -> Terminator_19/1
  Demux4/20 -> Terminator_20/1
  Demux4/21 -> Terminator_21/1
  Demux4/22 -> Terminator_22/1
  Demux4/23 -> Terminator_23/1
  Demux4/24 -> Terminator_24/1
  Demux4/25 -> Terminator_25/1
  Demux4/26 -> Terminator_26/1
